simulink model "SingleAgent_Drone"  (R2018b)
settings: Solver=VariableStepAuto  StartTime=0.0  StopTime=10  RelTol=1e-3
values from neighbouring files (symbols this model uses):
  p02 = zeros(SInfo2.n, 1)    [Parameters.m]
  q01 = zeros(SInfo1.n, 1)    [Parameters.m]
settings Model: Creator=oscar  LastModifiedBy=oscar

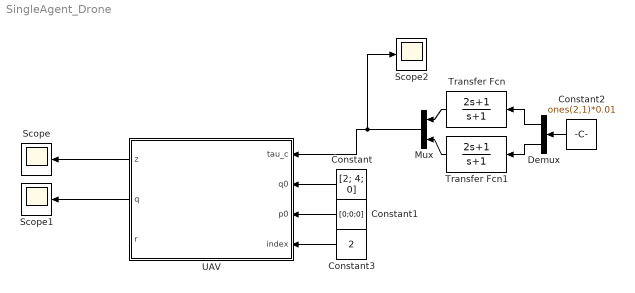
== system SingleAgent_Drone ==
  Constant : Constant  Value=[2; 4; 0]
  Constant1 : Constant  Value=[0;0;0]
  Constant2 : Constant  Value=ones(2,1)*0.01
  Constant3 : Constant  Value=2
  Demux : Demux  Outputs=2
  Mux : Mux  Inputs=2
  Scope : Scope
  Scope1 : Scope
  Scope2 : Scope
  Transfer Fcn : TransferFcn  Numerator=[2 1]  Denominator=[1 1]
  Transfer Fcn1 : TransferFcn  Numerator=[2 1]  Denominator=[1 1]
  UAV : Subsystem
  wires:
  Constant/1 -> UAV/2(q0)
  Constant1/1 -> UAV/3(p0)
  Constant2/1 -> Demux/1
  UAV/1(z) -> Scope/1
  UAV/2(q) -> Scope1/1
  Constant3/1 -> UAV/4(index)
  Transfer Fcn1/1 -> Mux/2
  Transfer Fcn/1 -> Mux/1
  Mux/1 -> Scope2/1, UAV/1(tau_c)
  Demux/1 -> Transfer Fcn/1
  Demux/2 -> Transfer Fcn1/1

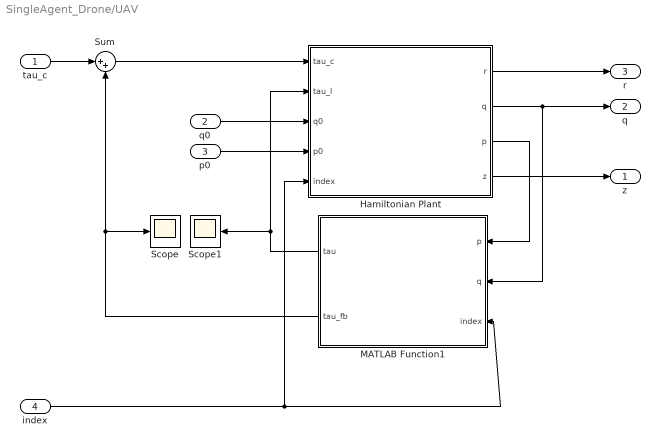
== system SingleAgent_Drone/UAV ==
  tau_c : Inport
  q0 : Inport  Port=2
  p0 : Inport  Port=3
  index : Inport  Port=4
  Hamiltonian Plant : Subsystem
  MATLAB Function1 : MATLAB Function  TreatAsAtomicUnit=on
  Scope : Scope
  Scope1 : Scope
  Sum : Sum  Inputs=|++
  z : Outport
  q : Outport  Port=2
  r : Outport  Port=3
  wires:
  MATLAB Function1/1(tau) -> Scope1/1, Hamiltonian Plant/2(tau_l)
  tau_c/1 -> Sum/1
  Hamiltonian Plant/3(p) -> MATLAB Function1/1(p)
  Hamiltonian Plant/2(q) -> q/1, MATLAB Function1/2(q)
  Hamiltonian Plant/4(z) -> z/1
  Hamiltonian Plant/1(r) -> r/1
  q0/1 -> Hamiltonian Plant/3(q0)
  p0/1 -> Hamiltonian Plant/4(p0)
  MATLAB Function1/2(tau_fb) -> Scope/1, Sum/2
  Sum/1 -> Hamiltonian Plant/1(tau_c)
  index/1 -> Hamiltonian Plant/5(index), MATLAB Function1/3(index)

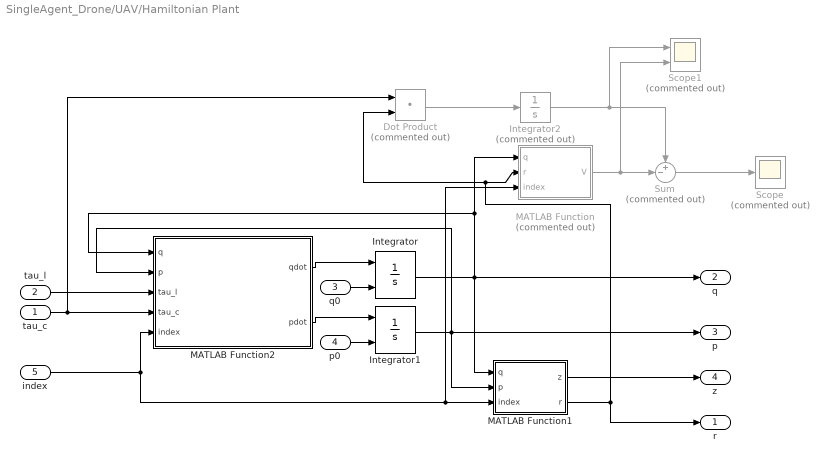
== system SingleAgent_Drone/UAV/Hamiltonian Plant ==
  tau_c : Inport
  tau_l : Inport  Port=2
  q0 : Inport  Port=3
  p0 : Inport  Port=4
  index : Inport  Port=5
  Dot Product : DotProduct  Commented=on  InputSameDT=on  OutDataTypeStr=Inherit: Inherit via internal rule
  Integrator : Integrator  InitialConditionSource=external  InitialCondition=q01
  Integrator1 : Integrator  InitialConditionSource=external  InitialCondition=p02
  Integrator2 : Integrator  Commented=on
  MATLAB Function : MATLAB Function  Commented=on  TreatAsAtomicUnit=on
  MATLAB Function1 : MATLAB Function  TreatAsAtomicUnit=on
  MATLAB Function2 : MATLAB Function  TreatAsAtomicUnit=on
  Scope : Scope  Commented=on
  Scope1 : Scope  Commented=on  NumInputPorts=2
  Sum : Sum  Commented=on  Inputs=+-|
  r : Outport
  q : Outport  Port=2
  p : Outport  Port=3
  z : Outport  Port=4
  wires:
  tau_l/1 -> MATLAB Function2/3(tau_l)
  MATLAB Function2/2(pdot) -> Integrator1/1
  Integrator1/1 -> MATLAB Function1/2(p), MATLAB Function2/2(p), p/1
  Integrator/1 -> MATLAB Function1/1(q), MATLAB Function/1(q), MATLAB Function2/1(q), q/1
  MATLAB Function2/1(qdot) -> Integrator/1
  p0/1 -> Integrator1/2
  tau_c/1 -> MATLAB Function2/4(tau_c), Dot Product/1
  q0/1 -> Integrator/2
  MATLAB Function/1(V) -> Scope1/2, Sum/2
  Dot Product/1 -> Integrator2/1
  Sum/1 -> Scope/1
  Integrator2/1 -> Scope1/1, Sum/1
  MATLAB Function1/1(z) -> z/1
  MATLAB Function1/2(r) -> MATLAB Function/2(r), Dot Product/2, r/1
  index/1 -> MATLAB Function/3(index), MATLAB Function1/3(index), MATLAB Function2/5(index)

== matlab function SingleAgent_Drone/UAV/Hamiltonian Plant/MATLAB Function1 ==
  data: q input; z output; p input; r output; index input
function [z, r] = toz(q, p, index)

    coder.extrinsic('UAV_z');
    z = zeros(2, 1);
    r = zeros(2, 1);    
    [z, r] = UAV_z(q, p, index);

== matlab function SingleAgent_Drone/UAV/Hamiltonian Plant/MATLAB Function ==
  data: q input; r input; index input; V output; Vr0 parameter
function V = fcn(q, r, index, Vr0)

%     coder.extrinsic('R_Validation');
%     V = 0;
%     [V] = R_Validation(q, r, index);
%     V = V - Vr0;
V = 0;
end

== matlab function SingleAgent_Drone/UAV/Hamiltonian Plant/MATLAB Function2 ==
  data: q input; qdot output; p input; tau_l input; pdot output; tau_c input; index input
function [qdot, pdot] = fcn(q, p, tau_l, tau_c, index)

    coder.extrinsic('UAV_Dynamics');
    qdot = zeros(3, 1);
    pdot = zeros(3, 1);
    [qdot, pdot] = UAV_Dynamics(q, p, tau_l, tau_c, index);

== matlab function SingleAgent_Drone/UAV/MATLAB Function1 ==
  data: p input; q input; tau output; tau_fb output; index input
function [tau, tau_fb] = LocalControl(p, q, index)
    

coder.extrinsic('UAV_Control');
tau = zeros(2, 1);
tau_fb = zeros(2, 1);
[tau, tau_fb] = UAV_Control(q, p, index);
